simulink subsystem "ElectricalCoolingSystemSSC"  (R2023b)
settings: Solver=VariableStepAuto  StartTime=0.0  StopTime=10.0  RelTol=1e-3
undefined symbols (not defined in the file): BattTempInit, Loop, One, Pass, pipe, pump, radiator, T_env, tank, ThrmBatt, ThrmBatt1, ThrmBatt2, ThrmBatt3, ThrmBatt4, ThrmEM, ThrmEM1, ThrmEM2, ThrmEM3, ThrmEM4, ThrmPwrE, valve
libraries: fl_lib x105, nesl_utility_internal x10, SimscapeFluids_lib x7, nesl_utility x1, sdl_lib x1
(part 3 of 3)

== system ElectricalCoolingSystemSSC/Cold Plate/One-Loop/Cooling Plate (Pack 1) ==
  Battery to plate conduction : fl_lib/Thermal/Thermal Elements/Conductive Heat Transfer  thermal_type=foundation.enum.ConstantVariableTabulated.Constant  wall_geometry=foundation.enum.ConductionWallGeometry.Planar  area=0.5*2 m^2  thickness=1 mm  d_in=0.05 m  d_out=0.1 m  L=1 m  th_cond_min=10 W/(K*m)  th_cond=205 W/(m*K)  th_cond_TLU=[413, 401, 392, 383, 371, 357, 342] W/(K*m)  temp_TLU=[200, 273, 400, 600, 800, 1000, 1200] K  T_specify=off  T_priority=None  T=0 K  T_nominal_specify=off  T_nominal_unit=K  T_nominal_value=1  Q_specify=off  Q_priority=None  Q=0 W  Q_nominal_specify=off  Q_nominal_unit=W  Q_nominal_value=1
  "Plate mass " : fl_lib/Thermal/Thermal Elements/Thermal Mass  mass_type=foundation.enum.constant_variable.constant  mass=10*2 kg  sp_heat=910 J/kg/K  mass_min=1e-6 kg  num_ports=foundation.enum.numPorts2.one  m_specify=off  m_priority=High  m=1 kg  m_nominal_specify=off  m_nominal_unit=kg  m_nominal_value=1  T_specify=on  T_priority=High  T=BattTempInit degC  T_nominal_specify=off  T_nominal_unit=K  T_nominal_value=1  Q_specify=off  Q_priority=None  Q=0 W  Q_nominal_specify=off  Q_nominal_unit=W  Q_nominal_value=1
  H1 : PMIOPort  Side=Left
  T1 : PMIOPort  Port=2  Side=Right
  connections:
  T1/RConn1 -- Battery to plate conduction/LConn1
  Battery to plate conduction/RConn1 -- H1/RConn1 -- "Plate mass "/LConn1

== system ElectricalCoolingSystemSSC/Cold Plate/One-Pass/Cooling Plate (Pack 1) ==
  Battery to plate conduction : fl_lib/Thermal/Thermal Elements/Conductive Heat Transfer  thermal_type=foundation.enum.ConstantVariableTabulated.Constant  wall_geometry=foundation.enum.ConductionWallGeometry.Planar  area=0.5*2 m^2  thickness=1 mm  d_in=0.05 m  d_out=0.1 m  L=1 m  th_cond_min=10 W/(K*m)  th_cond=205 W/(m*K)  th_cond_TLU=[413, 401, 392, 383, 371, 357, 342] W/(K*m)  temp_TLU=[200, 273, 400, 600, 800, 1000, 1200] K  T_specify=off  T_priority=None  T=0 K  T_nominal_specify=off  T_nominal_unit=K  T_nominal_value=1  Q_specify=off  Q_priority=None  Q=0 W  Q_nominal_specify=off  Q_nominal_unit=W  Q_nominal_value=1
  "Plate mass " : fl_lib/Thermal/Thermal Elements/Thermal Mass  mass_type=foundation.enum.constant_variable.constant  mass=10*2 kg  sp_heat=910 J/kg/K  mass_min=1e-6 kg  num_ports=foundation.enum.numPorts2.one  m_specify=off  m_priority=High  m=1 kg  m_nominal_specify=off  m_nominal_unit=kg  m_nominal_value=1  T_specify=on  T_priority=High  T=BattTempInit degC  T_nominal_specify=off  T_nominal_unit=K  T_nominal_value=1  Q_specify=off  Q_priority=None  Q=0 W  Q_nominal_specify=off  Q_nominal_unit=W  Q_nominal_value=1
  H1 : PMIOPort  Side=Left
  T1 : PMIOPort  Port=2  Side=Right
  connections:
  T1/RConn1 -- Battery to plate conduction/LConn1
  "Plate mass "/LConn1 -- H1/RConn1 -- Battery to plate conduction/RConn1

== system ElectricalCoolingSystemSSC/Cold Plate/One-Pass/Cooling Plate (Pack 2) ==
  Battery to plate conduction : fl_lib/Thermal/Thermal Elements/Conductive Heat Transfer  thermal_type=foundation.enum.ConstantVariableTabulated.Constant  wall_geometry=foundation.enum.ConductionWallGeometry.Planar  area=0.5*2 m^2  thickness=1 mm  d_in=0.05 m  d_out=0.1 m  L=1 m  th_cond_min=10 W/(K*m)  th_cond=205 W/(m*K)  th_cond_TLU=[413, 401, 392, 383, 371, 357, 342] W/(K*m)  temp_TLU=[200, 273, 400, 600, 800, 1000, 1200] K  T_specify=off  T_priority=None  T=0 K  T_nominal_specify=off  T_nominal_unit=K  T_nominal_value=1  Q_specify=off  Q_priority=None  Q=0 W  Q_nominal_specify=off  Q_nominal_unit=W  Q_nominal_value=1
  "Plate mass " : fl_lib/Thermal/Thermal Elements/Thermal Mass  mass_type=foundation.enum.constant_variable.constant  mass=10*2 kg  sp_heat=910 J/kg/K  mass_min=1e-6 kg  num_ports=foundation.enum.numPorts2.one  m_specify=off  m_priority=High  m=1 kg  m_nominal_specify=off  m_nominal_unit=kg  m_nominal_value=1  T_specify=on  T_priority=High  T=BattTempInit degC  T_nominal_specify=off  T_nominal_unit=K  T_nominal_value=1  Q_specify=off  Q_priority=None  Q=0 W  Q_nominal_specify=off  Q_nominal_unit=W  Q_nominal_value=1
  H1 : PMIOPort  Side=Left
  T2 : PMIOPort  Port=2  Side=Right
  connections:
  T2/RConn1 -- Battery to plate conduction/LConn1
  "Plate mass "/LConn1 -- H1/RConn1 -- Battery to plate conduction/RConn1

== system ElectricalCoolingSystemSSC/Cold Plate/One-Pass/Cooling Plate (Pack 3) ==
  Battery to plate conduction : fl_lib/Thermal/Thermal Elements/Conductive Heat Transfer  thermal_type=foundation.enum.ConstantVariableTabulated.Constant  wall_geometry=foundation.enum.ConductionWallGeometry.Planar  area=0.5*2 m^2  thickness=1 mm  d_in=0.05 m  d_out=0.1 m  L=1 m  th_cond_min=10 W/(K*m)  th_cond=205 W/(m*K)  th_cond_TLU=[413, 401, 392, 383, 371, 357, 342] W/(K*m)  temp_TLU=[200, 273, 400, 600, 800, 1000, 1200] K  T_specify=off  T_priority=None  T=0 K  T_nominal_specify=off  T_nominal_unit=K  T_nominal_value=1  Q_specify=off  Q_priority=None  Q=0 W  Q_nominal_specify=off  Q_nominal_unit=W  Q_nominal_value=1
  "Plate mass " : fl_lib/Thermal/Thermal Elements/Thermal Mass  mass_type=foundation.enum.constant_variable.constant  mass=10*2 kg  sp_heat=910 J/kg/K  mass_min=1e-6 kg  num_ports=foundation.enum.numPorts2.one  m_specify=off  m_priority=High  m=1 kg  m_nominal_specify=off  m_nominal_unit=kg  m_nominal_value=1  T_specify=on  T_priority=High  T=BattTempInit degC  T_nominal_specify=off  T_nominal_unit=K  T_nominal_value=1  Q_specify=off  Q_priority=None  Q=0 W  Q_nominal_specify=off  Q_nominal_unit=W  Q_nominal_value=1
  H1 : PMIOPort  Side=Left
  T3 : PMIOPort  Port=2  Side=Right
  connections:
  T3/RConn1 -- Battery to plate conduction/LConn1
  Battery to plate conduction/RConn1 -- H1/RConn1 -- "Plate mass "/LConn1

== system ElectricalCoolingSystemSSC/Cold Plate/One-Pass/Cooling Plate (Pack 4) ==
  Battery to plate conduction : fl_lib/Thermal/Thermal Elements/Conductive Heat Transfer  thermal_type=foundation.enum.ConstantVariableTabulated.Constant  wall_geometry=foundation.enum.ConductionWallGeometry.Planar  area=0.5*2 m^2  thickness=1 mm  d_in=0.05 m  d_out=0.1 m  L=1 m  th_cond_min=10 W/(K*m)  th_cond=205 W/(m*K)  th_cond_TLU=[413, 401, 392, 383, 371, 357, 342] W/(K*m)  temp_TLU=[200, 273, 400, 600, 800, 1000, 1200] K  T_specify=off  T_priority=None  T=0 K  T_nominal_specify=off  T_nominal_unit=K  T_nominal_value=1  Q_specify=off  Q_priority=None  Q=0 W  Q_nominal_specify=off  Q_nominal_unit=W  Q_nominal_value=1
  "Plate mass " : fl_lib/Thermal/Thermal Elements/Thermal Mass  mass_type=foundation.enum.constant_variable.constant  mass=10*2 kg  sp_heat=910 J/kg/K  mass_min=1e-6 kg  num_ports=foundation.enum.numPorts2.one  m_specify=off  m_priority=High  m=1 kg  m_nominal_specify=off  m_nominal_unit=kg  m_nominal_value=1  T_specify=on  T_priority=High  T=BattTempInit degC  T_nominal_specify=off  T_nominal_unit=K  T_nominal_value=1  Q_specify=off  Q_priority=None  Q=0 W  Q_nominal_specify=off  Q_nominal_unit=W  Q_nominal_value=1
  H1 : PMIOPort  Side=Left
  T4 : PMIOPort  Port=2  Side=Right
  connections:
  T4/RConn1 -- Battery to plate conduction/LConn1
  "Plate mass "/LConn1 -- H1/RConn1 -- Battery to plate conduction/RConn1

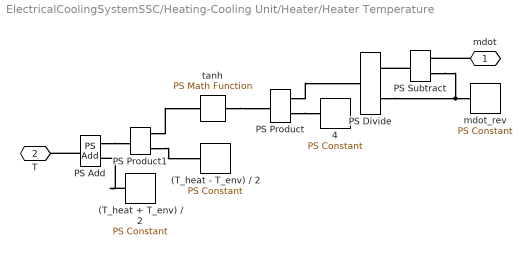
== system ElectricalCoolingSystemSSC/Heating-Cooling Unit/Heater/Heater Temperature ==
  (T_heat + T_env) / 2 : fl_lib/Physical Signals/Sources/PS Constant  constant=(T_heat +T_env + 273.15)/2 K
  (T_heat - T_env) / 2 : fl_lib/Physical Signals/Sources/PS Constant  constant=(T_heat - T_env - 273.15)/2 K
  4 : fl_lib/Physical Signals/Sources/PS Constant  constant=4
  PS Add : fl_lib/Physical Signals/Functions/PS Add
  PS Divide : fl_lib/Physical Signals/Functions/PS Divide
  PS Product : fl_lib/Physical Signals/Functions/PS Product
  PS Product1 : fl_lib/Physical Signals/Functions/PS Product
  PS Subtract : fl_lib/Physical Signals/Functions/PS Subtract
  mdot_rev : fl_lib/Physical Signals/Sources/PS Constant  constant=mdot_rev kg/s
  tanh : fl_lib/Physical Signals/Functions/PS Math Function  fcn_choice=foundation.enum.math_function.tanh  v=1
  mdot : PMIOPort  Side=Left
  T : PMIOPort  Port=2  Side=Right
  connections:
  PS Add/RConn1 -- T/RConn1
  tanh/LConn1 -- PS Product/RConn1
  PS Divide/LConn2 -- PS Subtract/LConn2 -- mdot_rev/RConn1
  PS Product/LConn2 -- 4/RConn1
  PS Add/LConn1 -- PS Product1/RConn1
  PS Subtract/RConn1 -- PS Divide/LConn1
  PS Product1/LConn2 -- (T_heat - T_env) / 2/RConn1
  PS Product1/LConn1 -- tanh/RConn1
  PS Product/LConn1 -- PS Divide/RConn1
  (T_heat + T_env) / 2/RConn1 -- PS Add/LConn2
  mdot/RConn1 -- PS Subtract/LConn1

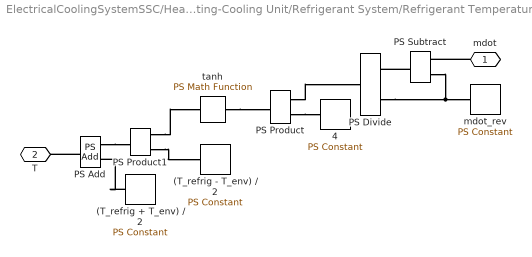
== system ElectricalCoolingSystemSSC/Heating-Cooling Unit/Refrigerant System/Refrigerant Temperature ==
  (T_refrig + T_env) / 2 : fl_lib/Physical Signals/Sources/PS Constant  constant=(T_refrig+T_env+273.15)/2 K
  (T_refrig - T_env) / 2 : fl_lib/Physical Signals/Sources/PS Constant  constant=(T_refrig-T_env-273.15)/2 K
  4 : fl_lib/Physical Signals/Sources/PS Constant  constant=4
  PS Add : fl_lib/Physical Signals/Functions/PS Add
  PS Divide : fl_lib/Physical Signals/Functions/PS Divide
  PS Product : fl_lib/Physical Signals/Functions/PS Product
  PS Product1 : fl_lib/Physical Signals/Functions/PS Product
  PS Subtract : fl_lib/Physical Signals/Functions/PS Subtract
  mdot_rev : fl_lib/Physical Signals/Sources/PS Constant  constant=mdot_rev kg/s
  tanh : fl_lib/Physical Signals/Functions/PS Math Function  fcn_choice=foundation.enum.math_function.tanh  v=1
  mdot : PMIOPort  Side=Left
  T : PMIOPort  Port=2  Side=Right
  connections:
  tanh/LConn1 -- PS Product/RConn1
  PS Product/LConn1 -- PS Divide/RConn1
  (T_refrig + T_env) / 2/RConn1 -- PS Add/LConn2
  PS Divide/LConn2 -- PS Subtract/LConn2 -- mdot_rev/RConn1
  PS Add/RConn1 -- T/RConn1
  PS Add/LConn1 -- PS Product1/RConn1
  PS Product1/LConn1 -- tanh/RConn1
  PS Product/LConn2 -- 4/RConn1
  PS Subtract/RConn1 -- PS Divide/LConn1
  PS Product1/LConn2 -- (T_refrig - T_env) / 2/RConn1
  mdot/RConn1 -- PS Subtract/LConn1
